simulink model "Ex_09_PD_ClosedLoopDOB_compat"  (Simulink 8.7)
settings: Solver=VariableStepAuto  SolverMode=SingleTasking  StartTime=0.0  StopTime=t_max  FixedStep=jointObj.Ts/10  RelTol=1e-3
values from neighbouring files (symbols this model uses):
  t_max = f_max    (= 100)    [Ex_00_example_config.m]
libraries: simulink x1, cjt_library_models x1, cjt_library_controllers x1
settings Model: Creator=joern  LastModifiedBy=J�rn
settings DataIOCC: LimitDataPoints=off
settings DebuggingCC: UnderspecifiedInitializationDetection=Simplified  MergeDetectMultiDrivingBlocksExec=error  SolverPrmCheckMsg=warning
settings ConfigComp: CovModelRefEnable=off  CovSFcnEnable=off

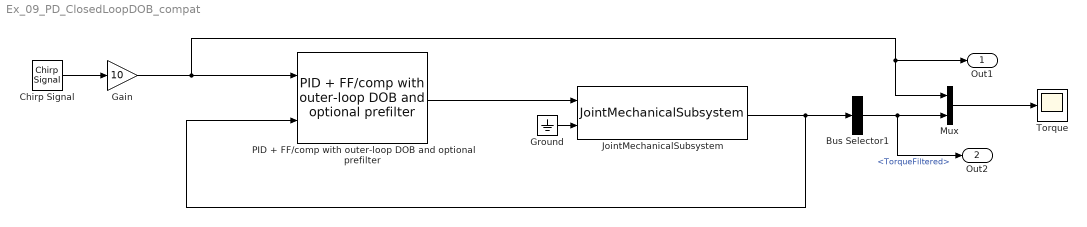
== system Ex_09_PD_ClosedLoopDOB_compat ==
  Bus Selector1 : BusSelector  OutputSignals=TorqueFiltered
  Chirp Signal : simulink/Sources/Chirp Signal  f1=f_min  T=t_max  f2=f_max
  Gain : Gain  Gain=10
  Ground : Ground
  JointMechanicalSubsystem : cjt_library_models/Joint models/JointMechanicalSubsystem  jointObj=jointObj  fc_vel=1000  fc_torque=1000  input_delay=0  output_delay=1  quantize=on  quantize_bits=19  input_noise_enabled=on  output_noise_enabled=on  var_u=0.12^2  var_y=1.8e-10
  Mux : Mux  Inputs=2
  PID + FF/comp with outer-loop DOB and optional prefilter : cjt_library_controllers/Controllers/PID + FF//comp with outer-loop DOB and optional prefilter  jointObj=jointObj  Kp=0.1  Ki=0  Kd=0.001  N=2*pi*200  ff_comp_switch=Feed-forward  DOB_enable_switch=On  premult_enable_switch=Off  loadData=off  modelFname=DOB_results.mat  f_c_FF=50  f_c_DOB=80
  Torque : Scope
  Out1 : Outport
  Out2 : Outport  Port=2
  wires:
  Mux/1 -> Torque/1
  Ground/1 -> JointMechanicalSubsystem/2
  JointMechanicalSubsystem/1 -> PID + FF/comp with outer-loop DOB and optional prefilter/2, Bus Selector1/1
  PID + FF/comp with outer-loop DOB and optional prefilter/1 -> JointMechanicalSubsystem/1
  Chirp Signal/1 -> Gain/1
  Bus Selector1/1 -> Out2/1, Mux/2  "<TorqueFiltered>"
  Gain/1 -> PID + FF/comp with outer-loop DOB and optional prefilter/1, Out1/1, Mux/1
